simulink model "Fan_Hysteresis_Model"  (R2025a)
settings: Solver=VariableStepAuto  StartTime=0.0  StopTime=10.0  RelTol=1e-3
libraries: simulink x2
settings Model: Creator=mahij  LastModifiedBy=mahij

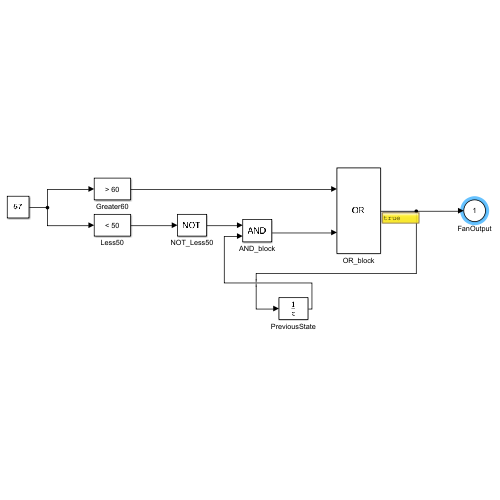
[thumbnail: Simulink's stored preview of the top-level diagram]
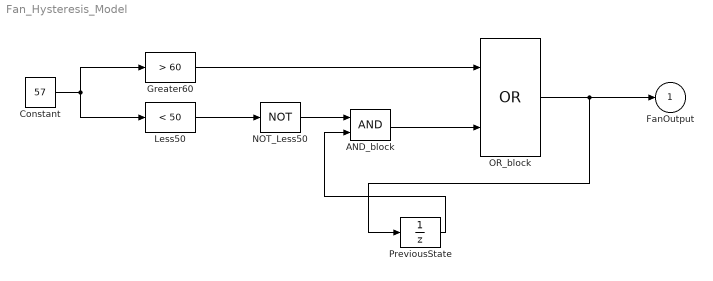
== system Fan_Hysteresis_Model ==
  AND_block : Logic  AllPortsSameDT=off  OutDataTypeStr=boolean
  Constant : Constant  Value=57
  Greater60 : simulink/Logic and Bit Operations/Compare To Constant  relop=>  const=60  OutDataTypeStr=boolean
  Less50 : simulink/Logic and Bit Operations/Compare To Constant  relop=<  const=50  OutDataTypeStr=boolean
  NOT_Less50 : Logic  Operator=NOT  AllPortsSameDT=off  OutDataTypeStr=boolean
  OR_block : Logic  Operator=OR  AllPortsSameDT=off  OutDataTypeStr=boolean
  PreviousState : UnitDelay  SampleTime=-1  HasFrameUpgradeWarning=on
  FanOutput : Outport
  wires:
  Constant/1 -> Greater60/1, Less50/1
  Less50/1 -> NOT_Less50/1
  NOT_Less50/1 -> AND_block/1
  PreviousState/1 -> AND_block/2
  Greater60/1 -> OR_block/1
  AND_block/1 -> OR_block/2
  OR_block/1 -> PreviousState/1, FanOutput/1
